simulink model "basic_charging_arm"  (R2022b)
settings: Solver=VariableStepAuto  StartTime=0.0  StopTime=100  RelTol=1e-3
values from neighbouring files (symbols this model uses):
  X = zeros(3,1)    [fk.m]
undefined symbols (not defined in the file or in its folder): Y, Z
libraries: fl_lib x64, fl_ps_legacy_lib x32, nesl_utility x25, sm_lib x24, simulink_extras x8, ee_lib x8, simulink x4, slpidlib x4, robotcorelib x1, robotmaniplib x1
(part 3 of 3)

== system basic_charging_arm/JOINT2/Controller/Speed/Step Rate and Direction/IC Analog Output REV ==
  SL : Inport
  Controlled Voltage Source : fl_lib/Electrical/Electrical Sources/Controlled Voltage Source
  ERef : fl_lib/Electrical/Electrical Elements/Electrical Reference
  Simulink-PS Converter : nesl_utility/Simulink-PS Converter  PhysicalDomain=network_engine_domain  SubClassName=ps_input  LeftPortType=input  RightPortType=output  PseudoPeriodic=off  Frequencies=[]  NoiseDistribution=none  NoiseParameters=[]  Unit=V  AffineConversion=off  FilteringAndDerivatives=zero  SimscapeFilterOrder=1  InputFilterTimeConstant=.001  UdotUserProvided=0
  V : PMIOPort  Side=Right
  wires:
  SL/1 -> Simulink-PS Converter/1
  connections:
  Simulink-PS Converter/RConn1 -- Controlled Voltage Source/RConn1
  V/RConn1 -- Controlled Voltage Source/LConn1
  ERef/LConn1 -- Controlled Voltage Source/RConn2

== system basic_charging_arm/JOINT2/Controller/Speed/Step Rate and Direction/IC Analog Output Vref ==
  SL : Inport
  Controlled Voltage Source : fl_lib/Electrical/Electrical Sources/Controlled Voltage Source
  ERef : fl_lib/Electrical/Electrical Elements/Electrical Reference
  Simulink-PS Converter : nesl_utility/Simulink-PS Converter  PhysicalDomain=network_engine_domain  SubClassName=ps_input  LeftPortType=input  RightPortType=output  PseudoPeriodic=off  Frequencies=[]  NoiseDistribution=none  NoiseParameters=[]  Unit=V  AffineConversion=off  FilteringAndDerivatives=zero  SimscapeFilterOrder=1  InputFilterTimeConstant=.001  UdotUserProvided=0
  V : PMIOPort  Side=Right
  wires:
  SL/1 -> Simulink-PS Converter/1
  connections:
  ERef/LConn1 -- Controlled Voltage Source/RConn2
  V/RConn1 -- Controlled Voltage Source/LConn1
  Simulink-PS Converter/RConn1 -- Controlled Voltage Source/RConn1

== system basic_charging_arm/JOINT3/Controller/Speed/Step Rate and Direction/IC Analog Output REV ==
  SL : Inport
  Controlled Voltage Source : fl_lib/Electrical/Electrical Sources/Controlled Voltage Source
  ERef : fl_lib/Electrical/Electrical Elements/Electrical Reference
  Simulink-PS Converter : nesl_utility/Simulink-PS Converter  PhysicalDomain=network_engine_domain  SubClassName=ps_input  LeftPortType=input  RightPortType=output  PseudoPeriodic=off  Frequencies=[]  NoiseDistribution=none  NoiseParameters=[]  Unit=V  AffineConversion=off  FilteringAndDerivatives=zero  SimscapeFilterOrder=1  InputFilterTimeConstant=.001  UdotUserProvided=0
  V : PMIOPort  Side=Right
  wires:
  SL/1 -> Simulink-PS Converter/1
  connections:
  ERef/LConn1 -- Controlled Voltage Source/RConn2
  V/RConn1 -- Controlled Voltage Source/LConn1
  Simulink-PS Converter/RConn1 -- Controlled Voltage Source/RConn1

== system basic_charging_arm/JOINT3/Controller/Speed/Step Rate and Direction/IC Analog Output Vref ==
  SL : Inport
  Controlled Voltage Source : fl_lib/Electrical/Electrical Sources/Controlled Voltage Source
  ERef : fl_lib/Electrical/Electrical Elements/Electrical Reference
  Simulink-PS Converter : nesl_utility/Simulink-PS Converter  PhysicalDomain=network_engine_domain  SubClassName=ps_input  LeftPortType=input  RightPortType=output  PseudoPeriodic=off  Frequencies=[]  NoiseDistribution=none  NoiseParameters=[]  Unit=V  AffineConversion=off  FilteringAndDerivatives=zero  SimscapeFilterOrder=1  InputFilterTimeConstant=.001  UdotUserProvided=0
  V : PMIOPort  Side=Right
  wires:
  SL/1 -> Simulink-PS Converter/1
  connections:
  Simulink-PS Converter/RConn1 -- Controlled Voltage Source/RConn1
  V/RConn1 -- Controlled Voltage Source/LConn1
  ERef/LConn1 -- Controlled Voltage Source/RConn2

== system basic_charging_arm/JOINT4/Controller/Speed/Step Rate and Direction/IC Analog Output REV ==
  SL : Inport
  Controlled Voltage Source : fl_lib/Electrical/Electrical Sources/Controlled Voltage Source
  ERef : fl_lib/Electrical/Electrical Elements/Electrical Reference
  Simulink-PS Converter : nesl_utility/Simulink-PS Converter  PhysicalDomain=network_engine_domain  SubClassName=ps_input  LeftPortType=input  RightPortType=output  PseudoPeriodic=off  Frequencies=[]  NoiseDistribution=none  NoiseParameters=[]  Unit=V  AffineConversion=off  FilteringAndDerivatives=zero  SimscapeFilterOrder=1  InputFilterTimeConstant=.001  UdotUserProvided=0
  V : PMIOPort  Side=Right
  wires:
  SL/1 -> Simulink-PS Converter/1
  connections:
  Simulink-PS Converter/RConn1 -- Controlled Voltage Source/RConn1
  V/RConn1 -- Controlled Voltage Source/LConn1
  ERef/LConn1 -- Controlled Voltage Source/RConn2

== system basic_charging_arm/JOINT4/Controller/Speed/Step Rate and Direction/IC Analog Output Vref ==
  SL : Inport
  Controlled Voltage Source : fl_lib/Electrical/Electrical Sources/Controlled Voltage Source
  ERef : fl_lib/Electrical/Electrical Elements/Electrical Reference
  Simulink-PS Converter : nesl_utility/Simulink-PS Converter  PhysicalDomain=network_engine_domain  SubClassName=ps_input  LeftPortType=input  RightPortType=output  PseudoPeriodic=off  Frequencies=[]  NoiseDistribution=none  NoiseParameters=[]  Unit=V  AffineConversion=off  FilteringAndDerivatives=zero  SimscapeFilterOrder=1  InputFilterTimeConstant=.001  UdotUserProvided=0
  V : PMIOPort  Side=Right
  wires:
  SL/1 -> Simulink-PS Converter/1
  connections:
  ERef/LConn1 -- Controlled Voltage Source/RConn2
  V/RConn1 -- Controlled Voltage Source/LConn1
  Simulink-PS Converter/RConn1 -- Controlled Voltage Source/RConn1

== matlab function basic_charging_arm/update_joint_angles ==
  data: q1 input; q1 output; q2 input; q3 input; q4 input; X input; q2 output; q3 output; q4 output
function [q1,q2,q3,q4] = i_k(q1,q2,q3,q4,X)
    X_goal =  [0.11; 0.7; 0.96];  
    del_X = X_goal - X;
    
    tolerance = 0.001;
    if norm(del_X) > tolerance
        %calculating jacobian 
        j = zeros(3,4);
        q2=-q2;
        q3=-q3;
        q4=-q4;
        j(1,1) = (261*sin(q4)*(sin(q1)*sin(q2)*sin(q3) - cos(q2)*cos(q3)*sin(q1)))/1000 - (261*cos(q4)*(cos(q2)*sin(q1)*sin(q3) + cos(q3)*sin(q1)*sin(q2)))/1000 - (8*sin(q1)*sin(q2))/25 - (7*cos(q2)*sin(q1)*sin(q3))/20 - (7*cos(q3)*sin(q1)*sin(q2))/20;
        
        j(1,2) = (8*cos(q1)*cos(q2))/25 + (261*cos(q4)*(cos(q1)*cos(q2)*cos(q3) - cos(q1)*sin(q2)*sin(q3)))/1000 - (261*sin(q4)*(cos(q1)*cos(q2)*sin(q3) + cos(q1)*cos(q3)*sin(q2)))/1000 + (7*cos(q1)*cos(q2)*cos(q3))/20 - (7*cos(q1)*sin(q2)*sin(q3))/20;
        
        j(1,3) = (261*cos(q4)*(cos(q1)*cos(q2)*cos(q3) - cos(q1)*sin(q2)*sin(q3)))/1000 - (261*sin(q4)*(cos(q1)*cos(q2)*sin(q3) + cos(q1)*cos(q3)*sin(q2)))/1000 + (7*cos(q1)*cos(q2)*cos(q3))/20 - (7*cos(q1)*sin(q2)*sin(q3))/20;
        
        j(1,4) = (261*cos(q4)*(cos(q1)*cos(q2)*cos(q3) - cos(q1)*sin(q2)*sin(q3)))/1000 - (261*sin(q4)*(cos(q1)*cos(q2)*sin(q3) + cos(q1)*cos(q3)*sin(q2)))/1000;
        
        j(2,1) = (8*cos(q1)*sin(q2))/25 + (261*cos(q4)*(cos(q1)*cos(q2)*sin(q3) + cos(q1)*cos(q3)*sin(q2)))/1000 + (261*sin(q4)*(cos(q1)*cos(q2)*cos(q3) - cos(q1)*sin(q2)*sin(q3)))/1000 + (7*cos(q1)*cos(q2)*sin(q3))/20 + (7*cos(q1)*cos(q3)*sin(q2))/20;
        
        j(2,2) = (8*cos(q2)*sin(q1))/25 - (261*cos(q4)*(sin(q1)*sin(q2)*sin(q3) - cos(q2)*cos(q3)*sin(q1)))/1000 - (261*sin(q4)*(cos(q2)*sin(q1)*sin(q3) + cos(q3)*sin(q1)*sin(q2)))/1000 - (7*sin(q1)*sin(q2)*sin(q3))/20 + (7*cos(q2)*cos(q3)*sin(q1))/20;
        
        j(2,3) = (7*cos(q2)*cos(q3)*sin(q1))/20 - (261*sin(q4)*(cos(q2)*sin(q1)*sin(q3) + cos(q3)*sin(q1)*sin(q2)))/1000 - (7*sin(q1)*sin(q2)*sin(q3))/20 - (261*cos(q4)*(sin(q1)*sin(q2)*sin(q3) - cos(q2)*cos(q3)*sin(q1)))/1000;
        
        j(2,4) = -(261*cos(q4)*(sin(q1)*sin(q2)*sin(q3) - cos(q2)*cos(q3)*sin(q1)))/1000 - (261*sin(q4)*(cos(q2)*sin(q1)*sin(q3) + cos(q3)*sin(q1)*sin(q2)))/1000;
        
        j(3,1) = 0;
        
        j(3,2) = -(8*sin(q2))/25 - (7*cos(q2)*sin(q3))/20 - (7*cos(q3)*sin(q2))/20 - (261*cos(q4)*(cos(q2)*sin(q3) + cos(q3)*sin(q2)))/1000 - (261*sin(q4)*(cos(q2)*cos(q3) - sin(q2)*sin(q3)))/1000;
        
        j(3,3) = -(7*cos(q2)*sin(q3))/20 - (7*cos(q3)*sin(q2))/20 - (261*cos(q4)*(cos(q2)*sin(q3) + cos(q3)*sin(q2)))/1000 - (261*sin(q4)*(cos(q2)*cos(q3) - sin(q2)*sin(q3)))/1000;
        
        j(3,4) = -(261*cos(q4)*(cos(q2)*sin(q3) + cos(q3)*sin(q2)))/1000 - (261*sin(q4)*(cos(q2)*cos(q3) - sin(q2)*sin(q3)))/1000;
        q2=-q2;
        q3=-q3;
        q4=-q4;
               
        jpinv = pinv(j);
        del_Q = jpinv*del_X;
        K = 1;
        q1 = q1 + K* del_Q(1,1);
        q2 = q2 + K* del_Q(2,1);
        q3 = q3 + K* del_Q(3,1);
        q4 = q4 + K* del_Q(4,1);

        if (q2 > 1.39)
           q2 = 1.39;
        elseif (q2 < -1.39)
                q2 = -1.39;
        end

        if (q3 > 1.39)
           q3 = 1.39;
        elseif (q3 < -1.39)
                q3 = -1.39;
        end

        if (q4 > 1.39)
           q4 = 1.39;
        elseif (q4 < -1.39)
                q4 = -1.39;
        end
          
   
    else
        
    end

pause(1)
end
